simulink model "multi_rotor_sim"  (R2023b)
settings: Solver=ode4  StartTime=0.0  StopTime=inf  FixedStep=ST  RelTol=1e-3
values from neighbouring files (symbols this model uses):
  a0 = 0    [parameters.m]
  ASLOPE = 5.9    [parameters.m]
  Ax = 0.023    [parameters.m]
  Ay = 0.023    [parameters.m]
  Az = 0.106    [parameters.m]
  BLADES = 2    [parameters.m]
  BLCG = 0    [parameters.m]
  BLCP = 0    [parameters.m]
  BLH1 = b*sind(30)    [parameters.m]
  BLH2 = b    (= 0.275)    [parameters.m]
  BLH3 = b*sind(30)    [parameters.m]
  BLH4 = -b*sind(30)    [parameters.m]
  BLH5 = -b    (= -0.275)    [parameters.m]
  BLH6 = -b*sind(30)    [parameters.m]
  chi1 = 1    [parameters.m]
  chi2 = -1    [parameters.m]
  chi3 = 1    [parameters.m]
  chi4 = -1    [parameters.m]
  chi5 = 1    [parameters.m]
  chi6 = -1    [parameters.m]
  CHORD = 17.55e-3    (= 0.01755)    [parameters.m]
  CHORD75 = 21e-3    (= 0.021)    [parameters.m]
  dyn_viscosity = 17.89e-6    (= 1.789e-05)    [parameters.m]
  g0 = 9.80665    [parameters.m]
  href = 0    [parameters.m]
  k_ind = 1.35    [parameters.m]
  k_Omega = 14.92    [parameters.m]
  latref = 44.200626    [parameters.m]
  lonref = 12.063822    [parameters.m]
  m = 2.15    [parameters.m]
  MC_ATT_PITCH = 45*pi/180    (= 0.785398163397)    [parameters.m]
  MC_ATT_ROLL = 45*pi/180    (= 0.785398163397)    [parameters.m]
  MC_PITCH_P = 2    [parameters.m]
  MC_PITCHRATE_D = 0    [parameters.m]
  MC_PITCHRATE_I = 0.05    [parameters.m]
  MC_PITCHRATE_P = 0.09*3    (= 0.27)    [parameters.m]
  MC_RATE_PITCH = 500*pi/180    (= 8.72664625997)    [parameters.m]
  MC_RATE_ROLL = 500*pi/180    (= 8.72664625997)    [parameters.m]
  MC_RATE_YAW = 300*pi/180    (= 5.23598775598)    [parameters.m]
  MC_ROLL_P = 2    [parameters.m]
  MC_ROLLRATE_D = 0    [parameters.m]
  MC_ROLLRATE_I = 0.05    [parameters.m]
  MC_ROLLRATE_P = 0.09*3    (= 0.27)    [parameters.m]
  MC_VEL_FWD = 15    [parameters.m]
  MC_VEL_FWD_OPT = 0.5    [parameters.m]
  MC_VEL_LAT = 15    [parameters.m]
  MC_VEL_LAT_OPT = 0.5    [parameters.m]
  MC_VEL_VERT = 15    [parameters.m]
  MC_YAW_P = 0.55    [parameters.m]
  MC_YAWRATE_D = 0.05    [parameters.m]
  MC_YAWRATE_I = 0.02    [parameters.m]
  MC_YAWRATE_P = 0.15*3    (= 0.45)    [parameters.m]
  MPC_XY_VEL_D_ACC = 0.6    [parameters.m]
  MPC_XY_VEL_I_ACC = 0.8    [parameters.m]
  MPC_XY_VEL_P_ACC = 1.7    [parameters.m]
  MPC_Z_VEL_D_ACC = 0    [parameters.m]
  MPC_Z_VEL_I_ACC = 2    [parameters.m]
  MPC_Z_VEL_P_ACC = 4    [parameters.m]
  n = 0.6359    [parameters.m]
  p00 = 7.145e-2    (= 0.07145)    [parameters.m]
  p01 = 0.4377    [parameters.m]
  p02 = -10.13    [parameters.m]
  p10 = 1.259e-3    (= 0.001259)    [parameters.m]
  p11 = 1.284e-3    (= 0.001284)    [parameters.m]
  p20 = -7.513e-7    (= -7.513e-07)    [parameters.m]
  PWM_hover = (PWM_idle+PWM_max)/2    (= 1550)    [parameters.m]
  PWM_idle = 1100    [parameters.m]
  PWM_max = 2000    [parameters.m]
  ROTOR = 4*0.0254    (= 0.1016)    [parameters.m]
  ST = 0.01    [parameters.m]
  STACG = 0    [parameters.m]
  STACP = 0    [parameters.m]
  STAH1 = -b*cosd(30)    [parameters.m]
  STAH2 = 0    [parameters.m]
  STAH3 = b*cosd(30)    [parameters.m]
  STAH4 = b*cosd(30)    [parameters.m]
  STAH5 = 0    [parameters.m]
  STAH6 = -b*cosd(30)    [parameters.m]
  TERMINAL_SPEED = 0.5    [parameters.m]
  Theta0 = 45*pi/180    (= 0.785398163397)    [parameters.m]
  THETT = -38.0973*pi/180    (= -0.66492332112)    [parameters.m]
  wind_rate = [ 0 0 0 ]'    [parameters.m]
  wind_velocity_e = [ 0 0 0 ]'    [parameters.m]
  WLCG = -0.02    [parameters.m]
  WLCP = -0.08    [parameters.m]
  WLH1 = 32e-3    (= 0.032)    [parameters.m]
  WLH2 = 32e-3    (= 0.032)    [parameters.m]
  WLH3 = 32e-3    (= 0.032)    [parameters.m]
  WLH4 = 32e-3    (= 0.032)    [parameters.m]
  WLH5 = 32e-3    (= 0.032)    [parameters.m]
  WLH6 = 32e-3    (= 0.032)    [parameters.m]
undefined symbols (not defined in the file or in its folder): Earth, WGS84, X, Y, Z
libraries: sm_lib x258, slpidlib x36, nesl_utility x15, sharedtransform x13, aerolibutil x4, aerolibanimutils x3, sharedutil x2, sim3dlib x1, uavsim3dlib x1, shared6dof x1, aerolibtransform2 x1, aerolibatmos2 x1
(part 8 of 11)

== system multi_rotor_sim/3D_visualization/SIMECHANICS 3D SCENE/SimMechanics/MotorA/DCBL_Assembly_Clockwise_1_Top_1_RIGID ==
  Assem1DCBL_Assembly_Clockwise_1_Top_1_RIGID : Subsystem
  ReferenceFrame : sm_lib/Frames and Transforms/Reference Frame
  Transform : sm_lib/Frames and Transforms/Rigid Transform  TranslationMethod=Cartesian  TranslationStandardOffset=0  TranslationStandardOffsetUnits=mm  TranslationStandardAxis=+Z  TranslationCartesianOffset=[-1.7338900268269642e-14 5.4999999999999929 -2.252012665224854e-14]  TranslationCartesianOffsetUnits=mm  TranslationROffset=0  TranslationROffsetUnits=m  TranslationZOffset=0  TranslationZOffsetUnits=m  TranslationThetaOffset=0  TranslationThetaOffsetUnits=deg  RotationMethod=ArbitraryAxis  RotationAngleUnits=rad  RotationStandardAxis=+Z  RotationAngle=2.0943951023931957  RotationArbitraryAxis=[0.57735026918962584 -0.57735026918962573 0.57735026918962573]  FollAlignAxisA=+X  BaseAlignAxisA=+Y  FollAlignAxisB=+Y  BaseAlignAxisB=+Z  RotationSequenceAxes=FollowerAxes  RotationSequence=XYX  RotationSequenceAngles=[0 0 0]  RotationSequenceAnglesUnits=deg  RotationMatrix=[1 0 0; 0 1 0; 0 0 1]  Quaternion=[1 0 0 0]
  F : PMIOPort  Side=Left
  connections:
  ReferenceFrame/RConn1 -- Assem1DCBL_Assembly_Clockwise_1_Top_1_RIGID/LConn1 -- Transform/LConn1
  Transform/RConn1 -- F/RConn1

== system multi_rotor_sim/3D_visualization/SIMECHANICS 3D SCENE/SimMechanics/MotorB/DCBL_Assembly_CounterClockwise_2_Top_1_RIGID ==
  Assem2DCBL_Assembly_CounterClockwise_2_Top_1_RIGID : Subsystem
  ReferenceFrame : sm_lib/Frames and Transforms/Reference Frame
  Transform : sm_lib/Frames and Transforms/Rigid Transform  TranslationMethod=Cartesian  TranslationStandardOffset=0  TranslationStandardOffsetUnits=mm  TranslationStandardAxis=+Z  TranslationCartesianOffset=[5.4329271302963538e-14 5.5000000000000071 -8.6888702660306153e-14]  TranslationCartesianOffsetUnits=mm  TranslationROffset=0  TranslationROffsetUnits=m  TranslationZOffset=0  TranslationZOffsetUnits=m  TranslationThetaOffset=0  TranslationThetaOffsetUnits=deg  RotationMethod=ArbitraryAxis  RotationAngleUnits=rad  RotationStandardAxis=+Z  RotationAngle=2.0943951023931953  RotationArbitraryAxis=[0.57735026918962584 -0.57735026918962584 0.57735026918962584]  FollAlignAxisA=+X  BaseAlignAxisA=+Y  FollAlignAxisB=+Y  BaseAlignAxisB=+Z  RotationSequenceAxes=FollowerAxes  RotationSequence=XYX  RotationSequenceAngles=[0 0 0]  RotationSequenceAnglesUnits=deg  RotationMatrix=[1 0 0; 0 1 0; 0 0 1]  Quaternion=[1 0 0 0]
  F : PMIOPort  Side=Left
  connections:
  ReferenceFrame/RConn1 -- Assem2DCBL_Assembly_CounterClockwise_2_Top_1_RIGID/LConn1 -- Transform/LConn1
  Transform/RConn1 -- F/RConn1

== system multi_rotor_sim/3D_visualization/SIMECHANICS 3D SCENE/SimMechanics/MotorC/DCBL_Assembly_Clockwise_3_Top_1_RIGID ==
  Assem3DCBL_Assembly_Clockwise_3_Top_1_RIGID : Subsystem
  ReferenceFrame : sm_lib/Frames and Transforms/Reference Frame
  Transform : sm_lib/Frames and Transforms/Rigid Transform  TranslationMethod=Cartesian  TranslationStandardOffset=0  TranslationStandardOffsetUnits=mm  TranslationStandardAxis=+Z  TranslationCartesianOffset=[2.4199042072407481e-15 5.5000000000000071 -2.0095726513600741e-13]  TranslationCartesianOffsetUnits=mm  TranslationROffset=0  TranslationROffsetUnits=m  TranslationZOffset=0  TranslationZOffsetUnits=m  TranslationThetaOffset=0  TranslationThetaOffsetUnits=deg  RotationMethod=ArbitraryAxis  RotationAngleUnits=rad  RotationStandardAxis=+Z  RotationAngle=2.0943951023931953  RotationArbitraryAxis=[0.57735026918962584 -0.57735026918962584 0.57735026918962584]  FollAlignAxisA=+X  BaseAlignAxisA=+Y  FollAlignAxisB=+Y  BaseAlignAxisB=+Z  RotationSequenceAxes=FollowerAxes  RotationSequence=XYX  RotationSequenceAngles=[0 0 0]  RotationSequenceAnglesUnits=deg  RotationMatrix=[1 0 0; 0 1 0; 0 0 1]  Quaternion=[1 0 0 0]
  F : PMIOPort  Side=Left
  connections:
  ReferenceFrame/RConn1 -- Assem3DCBL_Assembly_Clockwise_3_Top_1_RIGID/LConn1 -- Transform/LConn1
  Transform/RConn1 -- F/RConn1

== system multi_rotor_sim/3D_visualization/SIMECHANICS 3D SCENE/SimMechanics/MotorD/DCBL_Assembly_CounterClockwise_4_Top_1_RIGID ==
  Assem4DCBL_Assembly_CounterClockwise_4_Top_1_RIGID : Subsystem
  ReferenceFrame : sm_lib/Frames and Transforms/Reference Frame
  Transform : sm_lib/Frames and Transforms/Rigid Transform  TranslationMethod=Cartesian  TranslationStandardOffset=0  TranslationStandardOffsetUnits=mm  TranslationStandardAxis=+Z  TranslationCartesianOffset=[2.4451512600426024e-14 5.5000000000000071 -1.4488516090253114e-14]  TranslationCartesianOffsetUnits=mm  TranslationROffset=0  TranslationROffsetUnits=m  TranslationZOffset=0  TranslationZOffsetUnits=m  TranslationThetaOffset=0  TranslationThetaOffsetUnits=deg  RotationMethod=ArbitraryAxis  RotationAngleUnits=rad  RotationStandardAxis=+Z  RotationAngle=2.0943951023931953  RotationArbitraryAxis=[0.57735026918962584 -0.57735026918962584 0.57735026918962584]  FollAlignAxisA=+X  BaseAlignAxisA=+Y  FollAlignAxisB=+Y  BaseAlignAxisB=+Z  RotationSequenceAxes=FollowerAxes  RotationSequence=XYX  RotationSequenceAngles=[0 0 0]  RotationSequenceAnglesUnits=deg  RotationMatrix=[1 0 0; 0 1 0; 0 0 1]  Quaternion=[1 0 0 0]
  F : PMIOPort  Side=Left
  connections:
  ReferenceFrame/RConn1 -- Assem4DCBL_Assembly_CounterClockwise_4_Top_1_RIGID/LConn1 -- Transform/LConn1
  Transform/RConn1 -- F/RConn1

== system multi_rotor_sim/3D_visualization/SIMECHANICS 3D SCENE/SimMechanics/Assembly_Quadrotor_NProp_1_RIGID/Assembly_Quadrotor_NoProp_1_RIGID/Arm1_DJI_F450_F550_Final_2_RIGID ==
  ReferenceFrame : sm_lib/Frames and Transforms/Reference Frame
  Solid : sm_lib/Body Elements/File Solid  ExtGeomFileName=Arm1-DJI F450 F550_Final_Default_sldprt.STL  UnitType=Custom  ExtGeomFileUnits=mm  StepReaderType=HEX  ExportConvexHullGeometry=off  InertiaType=Custom  Mass=0.040949498799243353  MassUnits=kg  CenterOfMass=[91.850565621128027 -9.6558313898433461 0.00059254732510302048]  CenterOfMassUnits=mm  MomentsOfInertia=[8.7857917451793011 208.43528107693191 210.30930845149899]  MomentsOfInertiaUnits=kg*mm^2  ProductsOfInertia=[0.00021379289914309399 -0.0030630676058125863 -5.324939120360261]  ProductsOfInertiaUnits=kg*mm^2  BasedOnType=Density  Density=1000  DensityUnits=kg/(m^3)  DoExposeReferenceFrame=on  SerializedFrames=<Frames/>  GraphicType=FromGeometry  MarkerShape=Sphere  MarkerSize=10  MarkerSizeUnits=m  GraphicVisPropType=SimpleVisualProperties  GraphicDiffuseColor=[1 1 1]  GraphicSpecularColor=[0.5 0.5 0.5 1.0]  GraphicAmbientColor=[0.15 0.15 0.15 1.0]  GraphicEmissiveColor=[0.0 0.0 0.0 1.0]  GraphicShininess=75  GraphicOpacity=1
  F : PMIOPort  Side=Left
  connections:
  Solid/RConn1 -- ReferenceFrame/RConn1 -- F/RConn1

== system multi_rotor_sim/3D_visualization/SIMECHANICS 3D SCENE/SimMechanics/Assembly_Quadrotor_NProp_1_RIGID/Assembly_Quadrotor_NoProp_1_RIGID/ArmRed1_DJI_F450_F550_Final_1_RIGID ==
  ReferenceFrame : sm_lib/Frames and Transforms/Reference Frame
  Solid : sm_lib/Body Elements/File Solid  ExtGeomFileName=ArmRed1-DJI F450 F550_Final_Default_sldprt.STL  UnitType=Custom  ExtGeomFileUnits=mm  StepReaderType=HEX  ExportConvexHullGeometry=off  InertiaType=Custom  Mass=0.040949498799243353  MassUnits=kg  CenterOfMass=[91.850565621128027 -9.6558313898433408 0.00059254732510311101]  CenterOfMassUnits=mm  MomentsOfInertia=[8.7857917451792904 208.43528107693191 210.30930845149899]  MomentsOfInertiaUnits=kg*mm^2  ProductsOfInertia=[0.00021379289914303225 -0.0030630676058125412 -5.3249391203602654]  ProductsOfInertiaUnits=kg*mm^2  BasedOnType=Density  Density=1000  DensityUnits=kg/(m^3)  DoExposeReferenceFrame=on  SerializedFrames=<Frames/>  GraphicType=FromGeometry  MarkerShape=Sphere  MarkerSize=10  MarkerSizeUnits=m  GraphicVisPropType=SimpleVisualProperties  GraphicDiffuseColor=[0.0 0.0 0.8]  GraphicSpecularColor=[0.5 0.5 0.5 1.0]  GraphicAmbientColor=[0.15 0.15 0.15 1.0]  GraphicEmissiveColor=[0.0 0.0 0.0 1.0]  GraphicShininess=75  GraphicOpacity=1
  F : PMIOPort  Side=Left
  connections:
  Solid/RConn1 -- ReferenceFrame/RConn1 -- F/RConn1

== system multi_rotor_sim/3D_visualization/SIMECHANICS 3D SCENE/SimMechanics/Assembly_Quadrotor_NProp_1_RIGID/Assembly_Quadrotor_NoProp_1_RIGID/ArmRed_DJI_F450_F550_Final_1_RIGID ==
  ReferenceFrame : sm_lib/Frames and Transforms/Reference Frame
  Solid : sm_lib/Body Elements/File Solid  ExtGeomFileName=ArmRed-DJI F450 F550_Final_Default_sldprt.STL  UnitType=Custom  ExtGeomFileUnits=mm  StepReaderType=HEX  ExportConvexHullGeometry=off  InertiaType=Custom  Mass=0.040949498799243353  MassUnits=kg  CenterOfMass=[91.850565621128027 -9.6558313898433461 0.00059254732510311101]  CenterOfMassUnits=mm  MomentsOfInertia=[8.7857917451793011 208.43528107693191 210.30930845149899]  MomentsOfInertiaUnits=kg*mm^2  ProductsOfInertia=[0.00021379289914314785 -0.0030630676058125421 -5.3249391203602672]  ProductsOfInertiaUnits=kg*mm^2  BasedOnType=Density  Density=1000  DensityUnits=kg/(m^3)  DoExposeReferenceFrame=on  SerializedFrames=<Frames/>  GraphicType=FromGeometry  MarkerShape=Sphere  MarkerSize=10  MarkerSizeUnits=m  GraphicVisPropType=SimpleVisualProperties  GraphicDiffuseColor=[0.0 0.0 0.8]  GraphicSpecularColor=[0.5 0.5 0.5 1.0]  GraphicAmbientColor=[0.15 0.15 0.15 1.0]  GraphicEmissiveColor=[0.0 0.0 0.0 1.0]  GraphicShininess=75  GraphicOpacity=1
  F : PMIOPort  Side=Left
  connections:
  Solid/RConn1 -- ReferenceFrame/RConn1 -- F/RConn1

== system multi_rotor_sim/3D_visualization/SIMECHANICS 3D SCENE/SimMechanics/Assembly_Quadrotor_NProp_1_RIGID/Assembly_Quadrotor_NoProp_1_RIGID/Arm_DJI_F450_F550_Final_1_RIGID ==
  ReferenceFrame : sm_lib/Frames and Transforms/Reference Frame
  Solid : sm_lib/Body Elements/File Solid  ExtGeomFileName=Arm-DJI F450 F550_Final_Default_sldprt.STL  UnitType=Custom  ExtGeomFileUnits=mm  StepReaderType=HEX  ExportConvexHullGeometry=off  InertiaType=Custom  Mass=0.040949498799243353  MassUnits=kg  CenterOfMass=[91.850565621128027 -9.6558313898433461 0.00059254732510274899]  CenterOfMassUnits=mm  MomentsOfInertia=[8.7857917451793011 208.43528107693191 210.30930845149899]  MomentsOfInertiaUnits=kg*mm^2  ProductsOfInertia=[0.00021379289914293239 -0.0030630676058130682 -5.324939120360269]  ProductsOfInertiaUnits=kg*mm^2  BasedOnType=Density  Density=1000  DensityUnits=kg/(m^3)  DoExposeReferenceFrame=on  SerializedFrames=<Frames/>  GraphicType=FromGeometry  MarkerShape=Sphere  MarkerSize=10  MarkerSizeUnits=m  GraphicVisPropType=SimpleVisualProperties  GraphicDiffuseColor=[1 1 1]  GraphicSpecularColor=[0.5 0.5 0.5 1.0]  GraphicAmbientColor=[0.15 0.15 0.15 1.0]  GraphicEmissiveColor=[0.0 0.0 0.0 1.0]  GraphicShininess=75  GraphicOpacity=1
  F : PMIOPort  Side=Left
  connections:
  Solid/RConn1 -- ReferenceFrame/RConn1 -- F/RConn1

== system multi_rotor_sim/3D_visualization/SIMECHANICS 3D SCENE/SimMechanics/Assembly_Quadrotor_NProp_1_RIGID/Assembly_Quadrotor_NoProp_1_RIGID/Bottom_board_DJI_F450_Final_1_RIGID ==
  ReferenceFrame : sm_lib/Frames and Transforms/Reference Frame
  Solid : sm_lib/Body Elements/File Solid  ExtGeomFileName=Bottom board-DJI F450_Final_Default_sldprt.STL  UnitType=Custom  ExtGeomFileUnits=mm  StepReaderType=HEX  ExportConvexHullGeometry=off  InertiaType=Custom  Mass=0.022402083580285712  MassUnits=kg  CenterOfMass=[0 4.8087280328776543e-11 0]  CenterOfMassUnits=mm  MomentsOfInertia=[17.621231604317398 65.326748791856005 47.714143483190369]  MomentsOfInertiaUnits=kg*mm^2  ProductsOfInertia=[0 0 0]  ProductsOfInertiaUnits=kg*mm^2  BasedOnType=Density  Density=1000  DensityUnits=kg/(m^3)  DoExposeReferenceFrame=on  SerializedFrames=<Frames/>  GraphicType=FromGeometry  MarkerShape=Sphere  MarkerSize=10  MarkerSizeUnits=m  GraphicVisPropType=SimpleVisualProperties  GraphicDiffuseColor=[0 0 0]  GraphicSpecularColor=[0.5 0.5 0.5 1.0]  GraphicAmbientColor=[0.15 0.15 0.15 1.0]  GraphicEmissiveColor=[0.0 0.0 0.0 1.0]  GraphicShininess=75  GraphicOpacity=1
  F : PMIOPort  Side=Left
  connections:
  Solid/RConn1 -- ReferenceFrame/RConn1 -- F/RConn1

== system multi_rotor_sim/3D_visualization/SIMECHANICS 3D SCENE/SimMechanics/Assembly_Quadrotor_NProp_1_RIGID/Assembly_Quadrotor_NoProp_1_RIGID/DCBL_Assembly_Clockwise_1_Bottom_1_RIGID ==
  De_DCBL_1_RIGID : Subsystem
  ReferenceFrame : sm_lib/Frames and Transforms/Reference Frame
  Transform : sm_lib/Frames and Transforms/Rigid Transform  TranslationMethod=None  TranslationStandardOffset=0  TranslationStandardOffsetUnits=m  TranslationStandardAxis=+Z  TranslationCartesianOffset=[0 0 0]  TranslationCartesianOffsetUnits=m  TranslationROffset=0  TranslationROffsetUnits=m  TranslationZOffset=0  TranslationZOffsetUnits=m  TranslationThetaOffset=0  TranslationThetaOffsetUnits=deg  RotationMethod=None  RotationAngleUnits=deg  RotationStandardAxis=+Z  RotationAngle=0  RotationArbitraryAxis=[0 0 1]  FollAlignAxisA=+X  BaseAlignAxisA=+Y  FollAlignAxisB=+Y  BaseAlignAxisB=+Z  RotationSequenceAxes=FollowerAxes  RotationSequence=XYX  RotationSequenceAngles=[0 0 0]  RotationSequenceAnglesUnits=deg  RotationMatrix=[1 0 0; 0 1 0; 0 0 1]  Quaternion=[1 0 0 0]
  Transform1 : sm_lib/Frames and Transforms/Rigid Transform  TranslationMethod=Cartesian  TranslationStandardOffset=0  TranslationStandardOffsetUnits=mm  TranslationStandardAxis=+Z  TranslationCartesianOffset=[159.70006653098284 35.76000000009617 159.70006653098039]  TranslationCartesianOffsetUnits=mm  TranslationROffset=0  TranslationROffsetUnits=m  TranslationZOffset=0  TranslationZOffsetUnits=m  TranslationThetaOffset=0  TranslationThetaOffsetUnits=deg  RotationMethod=ArbitraryAxis  RotationAngleUnits=rad  RotationStandardAxis=+Z  RotationAngle=0.78539816339744029  RotationArbitraryAxis=[0 -1 0]  FollAlignAxisA=+X  BaseAlignAxisA=+Y  FollAlignAxisB=+Y  BaseAlignAxisB=+Z  RotationSequenceAxes=FollowerAxes  RotationSequence=XYX  RotationSequenceAngles=[0 0 0]  RotationSequenceAnglesUnits=deg  RotationMatrix=[1 0 0; 0 1 0; 0 0 1]  Quaternion=[1 0 0 0]
  F : PMIOPort  Side=Right
  connections:
  De_DCBL_1_RIGID/LConn1 -- Transform/RConn1
  Transform/LConn1 -- ReferenceFrame/RConn1 -- Transform1/RConn1
  Transform1/LConn1 -- F/RConn1

== system multi_rotor_sim/3D_visualization/SIMECHANICS 3D SCENE/SimMechanics/Assembly_Quadrotor_NProp_1_RIGID/Assembly_Quadrotor_NoProp_1_RIGID/DCBL_Assembly_Clockwise_3_Bottom_1_RIGID ==
  De_DCBL_1_RIGID : Subsystem
  ReferenceFrame : sm_lib/Frames and Transforms/Reference Frame
  Transform : sm_lib/Frames and Transforms/Rigid Transform  TranslationMethod=None  TranslationStandardOffset=0  TranslationStandardOffsetUnits=m  TranslationStandardAxis=+Z  TranslationCartesianOffset=[0 0 0]  TranslationCartesianOffsetUnits=m  TranslationROffset=0  TranslationROffsetUnits=m  TranslationZOffset=0  TranslationZOffsetUnits=m  TranslationThetaOffset=0  TranslationThetaOffsetUnits=deg  RotationMethod=None  RotationAngleUnits=deg  RotationStandardAxis=+Z  RotationAngle=0  RotationArbitraryAxis=[0 0 1]  FollAlignAxisA=+X  BaseAlignAxisA=+Y  FollAlignAxisB=+Y  BaseAlignAxisB=+Z  RotationSequenceAxes=FollowerAxes  RotationSequence=XYX  RotationSequenceAngles=[0 0 0]  RotationSequenceAnglesUnits=deg  RotationMatrix=[1 0 0; 0 1 0; 0 0 1]  Quaternion=[1 0 0 0]
  Transform1 : sm_lib/Frames and Transforms/Rigid Transform  TranslationMethod=Cartesian  TranslationStandardOffset=0  TranslationStandardOffsetUnits=mm  TranslationStandardAxis=+Z  TranslationCartesianOffset=[-159.70006653098244 35.76000000009617 -159.70006653098108]  TranslationCartesianOffsetUnits=mm  TranslationROffset=0  TranslationROffsetUnits=m  TranslationZOffset=0  TranslationZOffsetUnits=m  TranslationThetaOffset=0  TranslationThetaOffsetUnits=deg  RotationMethod=ArbitraryAxis  RotationAngleUnits=rad  RotationStandardAxis=+Z  RotationAngle=0.78539816339744262  RotationArbitraryAxis=[0 -1 0]  FollAlignAxisA=+X  BaseAlignAxisA=+Y  FollAlignAxisB=+Y  BaseAlignAxisB=+Z  RotationSequenceAxes=FollowerAxes  RotationSequence=XYX  RotationSequenceAngles=[0 0 0]  RotationSequenceAnglesUnits=deg  RotationMatrix=[1 0 0; 0 1 0; 0 0 1]  Quaternion=[1 0 0 0]
  F : PMIOPort  Side=Right
  connections:
  De_DCBL_1_RIGID/LConn1 -- Transform/RConn1
  Transform/LConn1 -- ReferenceFrame/RConn1 -- Transform1/RConn1
  Transform1/LConn1 -- F/RConn1

== system multi_rotor_sim/3D_visualization/SIMECHANICS 3D SCENE/SimMechanics/Assembly_Quadrotor_NProp_1_RIGID/Assembly_Quadrotor_NoProp_1_RIGID/DCBL_Assembly_CounterClockwise_2_Bottom_1_RIGID ==
  De_DCBL_1_RIGID : Subsystem
  ReferenceFrame : sm_lib/Frames and Transforms/Reference Frame
  Transform : sm_lib/Frames and Transforms/Rigid Transform  TranslationMethod=None  TranslationStandardOffset=0  TranslationStandardOffsetUnits=m  TranslationStandardAxis=+Z  TranslationCartesianOffset=[0 0 0]  TranslationCartesianOffsetUnits=m  TranslationROffset=0  TranslationROffsetUnits=m  TranslationZOffset=0  TranslationZOffsetUnits=m  TranslationThetaOffset=0  TranslationThetaOffsetUnits=deg  RotationMethod=None  RotationAngleUnits=deg  RotationStandardAxis=+Z  RotationAngle=0  RotationArbitraryAxis=[0 0 1]  FollAlignAxisA=+X  BaseAlignAxisA=+Y  FollAlignAxisB=+Y  BaseAlignAxisB=+Z  RotationSequenceAxes=FollowerAxes  RotationSequence=XYX  RotationSequenceAngles=[0 0 0]  RotationSequenceAnglesUnits=deg  RotationMatrix=[1 0 0; 0 1 0; 0 0 1]  Quaternion=[1 0 0 0]
  Transform1 : sm_lib/Frames and Transforms/Rigid Transform  TranslationMethod=Cartesian  TranslationStandardOffset=0  TranslationStandardOffsetUnits=mm  TranslationStandardAxis=+Z  TranslationCartesianOffset=[159.7000665309815 35.76000000009617 -159.70006653098207]  TranslationCartesianOffsetUnits=mm  TranslationROffset=0  TranslationROffsetUnits=m  TranslationZOffset=0  TranslationZOffsetUnits=m  TranslationThetaOffset=0  TranslationThetaOffsetUnits=deg  RotationMethod=ArbitraryAxis  RotationAngleUnits=rad  RotationStandardAxis=+Z  RotationAngle=0.78539816339744961  RotationArbitraryAxis=[0 1 0]  FollAlignAxisA=+X  BaseAlignAxisA=+Y  FollAlignAxisB=+Y  BaseAlignAxisB=+Z  RotationSequenceAxes=FollowerAxes  RotationSequence=XYX  RotationSequenceAngles=[0 0 0]  RotationSequenceAnglesUnits=deg  RotationMatrix=[1 0 0; 0 1 0; 0 0 1]  Quaternion=[1 0 0 0]
  F : PMIOPort  Side=Right
  connections:
  De_DCBL_1_RIGID/LConn1 -- Transform/RConn1
  Transform/LConn1 -- ReferenceFrame/RConn1 -- Transform1/RConn1
  Transform1/LConn1 -- F/RConn1

== system multi_rotor_sim/3D_visualization/SIMECHANICS 3D SCENE/SimMechanics/Assembly_Quadrotor_NProp_1_RIGID/Assembly_Quadrotor_NoProp_1_RIGID/DCBL_Assembly_CounterClockwise_4_Bottom_1_RIGID ==
  De_DCBL_1_RIGID : Subsystem
  ReferenceFrame : sm_lib/Frames and Transforms/Reference Frame
  Transform : sm_lib/Frames and Transforms/Rigid Transform  TranslationMethod=None  TranslationStandardOffset=0  TranslationStandardOffsetUnits=m  TranslationStandardAxis=+Z  TranslationCartesianOffset=[0 0 0]  TranslationCartesianOffsetUnits=m  TranslationROffset=0  TranslationROffsetUnits=m  TranslationZOffset=0  TranslationZOffsetUnits=m  TranslationThetaOffset=0  TranslationThetaOffsetUnits=deg  RotationMethod=None  RotationAngleUnits=deg  RotationStandardAxis=+Z  RotationAngle=0  RotationArbitraryAxis=[0 0 1]  FollAlignAxisA=+X  BaseAlignAxisA=+Y  FollAlignAxisB=+Y  BaseAlignAxisB=+Z  RotationSequenceAxes=FollowerAxes  RotationSequence=XYX  RotationSequenceAngles=[0 0 0]  RotationSequenceAnglesUnits=deg  RotationMatrix=[1 0 0; 0 1 0; 0 0 1]  Quaternion=[1 0 0 0]
  Transform1 : sm_lib/Frames and Transforms/Rigid Transform  TranslationMethod=Cartesian  TranslationStandardOffset=0  TranslationStandardOffsetUnits=mm  TranslationStandardAxis=+Z  TranslationCartesianOffset=[-159.70006653098127 35.76000000009617 159.70006653098196]  TranslationCartesianOffsetUnits=mm  TranslationROffset=0  TranslationROffsetUnits=m  TranslationZOffset=0  TranslationZOffsetUnits=m  TranslationThetaOffset=0  TranslationThetaOffsetUnits=deg  RotationMethod=ArbitraryAxis  RotationAngleUnits=rad  RotationStandardAxis=+Z  RotationAngle=0.78539816339745094  RotationArbitraryAxis=[0 1 0]  FollAlignAxisA=+X  BaseAlignAxisA=+Y  FollAlignAxisB=+Y  BaseAlignAxisB=+Z  RotationSequenceAxes=FollowerAxes  RotationSequence=XYX  RotationSequenceAngles=[0 0 0]  RotationSequenceAnglesUnits=deg  RotationMatrix=[1 0 0; 0 1 0; 0 0 1]  Quaternion=[1 0 0 0]
  F : PMIOPort  Side=Right
  connections:
  De_DCBL_1_RIGID/LConn1 -- Transform/RConn1
  Transform/LConn1 -- ReferenceFrame/RConn1 -- Transform1/RConn1
  Transform1/LConn1 -- F/RConn1

== system multi_rotor_sim/3D_visualization/SIMECHANICS 3D SCENE/SimMechanics/Assembly_Quadrotor_NProp_1_RIGID/Assembly_Quadrotor_NoProp_1_RIGID/Top_board_DJI_F450_Final_1_RIGID ==
  ReferenceFrame : sm_lib/Frames and Transforms/Reference Frame
  Solid : sm_lib/Body Elements/File Solid  ExtGeomFileName=Top board-DJI F450_Final_Default_sldprt.STL  UnitType=Custom  ExtGeomFileUnits=mm  StepReaderType=HEX  ExportConvexHullGeometry=off  InertiaType=Custom  Mass=0.013626610836899209  MassUnits=kg  CenterOfMass=[0 0 0]  CenterOfMassUnits=mm  MomentsOfInertia=[11.678434060128888 23.780162168623775 12.106975262107815]  MomentsOfInertiaUnits=kg*mm^2  ProductsOfInertia=[0 0 0]  ProductsOfInertiaUnits=kg*mm^2  BasedOnType=Density  Density=1000  DensityUnits=kg/(m^3)  DoExposeReferenceFrame=on  SerializedFrames=<Frames/>  GraphicType=FromGeometry  MarkerShape=Sphere  MarkerSize=10  MarkerSizeUnits=m  GraphicVisPropType=SimpleVisualProperties  GraphicDiffuseColor=[0 0 0]  GraphicSpecularColor=[0.5 0.5 0.5 1.0]  GraphicAmbientColor=[0.15 0.15 0.15 1.0]  GraphicEmissiveColor=[0.0 0.0 0.0 1.0]  GraphicShininess=75  GraphicOpacity=1
  F : PMIOPort  Side=Left
  connections:
  Solid/RConn1 -- ReferenceFrame/RConn1 -- F/RConn1

== system multi_rotor_sim/3D_visualization/SIMECHANICS 3D SCENE/SimMechanics/Assembly_Quadrotor_NProp_1_RIGID/Assembly_Quadrotor_NoProp_1_RIGID/socket_head_cap_screw_iso_10_RIGID ==
  ReferenceFrame : sm_lib/Frames and Transforms/Reference Frame
  Solid : sm_lib/Body Elements/File Solid  ExtGeomFileName=socket head cap screw_iso_ISO 4762 M3 x 5 --- 5N_sldprt.STL  UnitType=Custom  ExtGeomFileUnits=mm  StepReaderType=HEX  ExportConvexHullGeometry=off  InertiaType=Custom  Mass=9.7562055451047927e-05  MassUnits=kg  CenterOfMass=[2.9922591429378405 0 0]  CenterOfMassUnits=mm  MomentsOfInertia=[0.00030067681878230242 0.000604867911685519 0.00060486791168551911]  MomentsOfInertiaUnits=kg*mm^2  ProductsOfInertia=[0 0 0]  ProductsOfInertiaUnits=kg*mm^2  BasedOnType=Density  Density=1000  DensityUnits=kg/(m^3)  DoExposeReferenceFrame=on  SerializedFrames=<Frames/>  GraphicType=FromGeometry  MarkerShape=Sphere  MarkerSize=10  MarkerSizeUnits=m  GraphicVisPropType=SimpleVisualProperties  GraphicDiffuseColor=[0.77647058823529413 0.75686274509803919 0.73725490196078436]  GraphicSpecularColor=[0.5 0.5 0.5 1.0]  GraphicAmbientColor=[0.15 0.15 0.15 1.0]  GraphicEmissiveColor=[0.0 0.0 0.0 1.0]  GraphicShininess=75  GraphicOpacity=1
  F : PMIOPort  Side=Left
  connections:
  Solid/RConn1 -- ReferenceFrame/RConn1 -- F/RConn1

== system multi_rotor_sim/3D_visualization/SIMECHANICS 3D SCENE/SimMechanics/Assembly_Quadrotor_NProp_1_RIGID/Assembly_Quadrotor_NoProp_1_RIGID/socket_head_cap_screw_iso_11_RIGID ==
  ReferenceFrame : sm_lib/Frames and Transforms/Reference Frame
  Solid : sm_lib/Body Elements/File Solid  ExtGeomFileName=socket head cap screw_iso_ISO 4762 M3 x 5 --- 5N_sldprt.STL  UnitType=Custom  ExtGeomFileUnits=mm  StepReaderType=HEX  ExportConvexHullGeometry=off  InertiaType=Custom  Mass=9.7562055451047927e-05  MassUnits=kg  CenterOfMass=[2.9922591429378405 0 0]  CenterOfMassUnits=mm  MomentsOfInertia=[0.00030067681878230242 0.000604867911685519 0.00060486791168551911]  MomentsOfInertiaUnits=kg*mm^2  ProductsOfInertia=[0 0 0]  ProductsOfInertiaUnits=kg*mm^2  BasedOnType=Density  Density=1000  DensityUnits=kg/(m^3)  DoExposeReferenceFrame=on  SerializedFrames=<Frames/>  GraphicType=FromGeometry  MarkerShape=Sphere  MarkerSize=10  MarkerSizeUnits=m  GraphicVisPropType=SimpleVisualProperties  GraphicDiffuseColor=[0.77647058823529413 0.75686274509803919 0.73725490196078436]  GraphicSpecularColor=[0.5 0.5 0.5 1.0]  GraphicAmbientColor=[0.15 0.15 0.15 1.0]  GraphicEmissiveColor=[0.0 0.0 0.0 1.0]  GraphicShininess=75  GraphicOpacity=1
  F : PMIOPort  Side=Left
  connections:
  Solid/RConn1 -- ReferenceFrame/RConn1 -- F/RConn1

== system multi_rotor_sim/3D_visualization/SIMECHANICS 3D SCENE/SimMechanics/Assembly_Quadrotor_NProp_1_RIGID/Assembly_Quadrotor_NoProp_1_RIGID/socket_head_cap_screw_iso_12_RIGID ==
  ReferenceFrame : sm_lib/Frames and Transforms/Reference Frame
  Solid : sm_lib/Body Elements/File Solid  ExtGeomFileName=socket head cap screw_iso_ISO 4762 M3 x 5 --- 5N_sldprt.STL  UnitType=Custom  ExtGeomFileUnits=mm  StepReaderType=HEX  ExportConvexHullGeometry=off  InertiaType=Custom  Mass=9.7562055451047927e-05  MassUnits=kg  CenterOfMass=[2.9922591429378405 0 0]  CenterOfMassUnits=mm  MomentsOfInertia=[0.00030067681878230242 0.000604867911685519 0.00060486791168551911]  MomentsOfInertiaUnits=kg*mm^2  ProductsOfInertia=[0 0 0]  ProductsOfInertiaUnits=kg*mm^2  BasedOnType=Density  Density=1000  DensityUnits=kg/(m^3)  DoExposeReferenceFrame=on  SerializedFrames=<Frames/>  GraphicType=FromGeometry  MarkerShape=Sphere  MarkerSize=10  MarkerSizeUnits=m  GraphicVisPropType=SimpleVisualProperties  GraphicDiffuseColor=[0.77647058823529413 0.75686274509803919 0.73725490196078436]  GraphicSpecularColor=[0.5 0.5 0.5 1.0]  GraphicAmbientColor=[0.15 0.15 0.15 1.0]  GraphicEmissiveColor=[0.0 0.0 0.0 1.0]  GraphicShininess=75  GraphicOpacity=1
  F : PMIOPort  Side=Left
  connections:
  Solid/RConn1 -- ReferenceFrame/RConn1 -- F/RConn1

== system multi_rotor_sim/3D_visualization/SIMECHANICS 3D SCENE/SimMechanics/Assembly_Quadrotor_NProp_1_RIGID/Assembly_Quadrotor_NoProp_1_RIGID/socket_head_cap_screw_iso_13_RIGID ==
  ReferenceFrame : sm_lib/Frames and Transforms/Reference Frame
  Solid : sm_lib/Body Elements/File Solid  ExtGeomFileName=socket head cap screw_iso_ISO 4762 M3 x 5 --- 5N_sldprt.STL  UnitType=Custom  ExtGeomFileUnits=mm  StepReaderType=HEX  ExportConvexHullGeometry=off  InertiaType=Custom  Mass=9.7562055451047927e-05  MassUnits=kg  CenterOfMass=[2.9922591429378405 0 0]  CenterOfMassUnits=mm  MomentsOfInertia=[0.00030067681878230242 0.000604867911685519 0.00060486791168551911]  MomentsOfInertiaUnits=kg*mm^2  ProductsOfInertia=[0 0 0]  ProductsOfInertiaUnits=kg*mm^2  BasedOnType=Density  Density=1000  DensityUnits=kg/(m^3)  DoExposeReferenceFrame=on  SerializedFrames=<Frames/>  GraphicType=FromGeometry  MarkerShape=Sphere  MarkerSize=10  MarkerSizeUnits=m  GraphicVisPropType=SimpleVisualProperties  GraphicDiffuseColor=[0.77647058823529413 0.75686274509803919 0.73725490196078436]  GraphicSpecularColor=[0.5 0.5 0.5 1.0]  GraphicAmbientColor=[0.15 0.15 0.15 1.0]  GraphicEmissiveColor=[0.0 0.0 0.0 1.0]  GraphicShininess=75  GraphicOpacity=1
  F : PMIOPort  Side=Left
  connections:
  Solid/RConn1 -- ReferenceFrame/RConn1 -- F/RConn1

== system multi_rotor_sim/3D_visualization/SIMECHANICS 3D SCENE/SimMechanics/Assembly_Quadrotor_NProp_1_RIGID/Assembly_Quadrotor_NoProp_1_RIGID/socket_head_cap_screw_iso_14_RIGID ==
  ReferenceFrame : sm_lib/Frames and Transforms/Reference Frame
  Solid : sm_lib/Body Elements/File Solid  ExtGeomFileName=socket head cap screw_iso_ISO 4762 M3 x 5 --- 5N_sldprt.STL  UnitType=Custom  ExtGeomFileUnits=mm  StepReaderType=HEX  ExportConvexHullGeometry=off  InertiaType=Custom  Mass=9.7562055451047927e-05  MassUnits=kg  CenterOfMass=[2.9922591429378405 0 0]  CenterOfMassUnits=mm  MomentsOfInertia=[0.00030067681878230242 0.000604867911685519 0.00060486791168551911]  MomentsOfInertiaUnits=kg*mm^2  ProductsOfInertia=[0 0 0]  ProductsOfInertiaUnits=kg*mm^2  BasedOnType=Density  Density=1000  DensityUnits=kg/(m^3)  DoExposeReferenceFrame=on  SerializedFrames=<Frames/>  GraphicType=FromGeometry  MarkerShape=Sphere  MarkerSize=10  MarkerSizeUnits=m  GraphicVisPropType=SimpleVisualProperties  GraphicDiffuseColor=[0.77647058823529413 0.75686274509803919 0.73725490196078436]  GraphicSpecularColor=[0.5 0.5 0.5 1.0]  GraphicAmbientColor=[0.15 0.15 0.15 1.0]  GraphicEmissiveColor=[0.0 0.0 0.0 1.0]  GraphicShininess=75  GraphicOpacity=1
  F : PMIOPort  Side=Left
  connections:
  Solid/RConn1 -- ReferenceFrame/RConn1 -- F/RConn1

== system multi_rotor_sim/3D_visualization/SIMECHANICS 3D SCENE/SimMechanics/Assembly_Quadrotor_NProp_1_RIGID/Assembly_Quadrotor_NoProp_1_RIGID/socket_head_cap_screw_iso_15_RIGID ==
  ReferenceFrame : sm_lib/Frames and Transforms/Reference Frame
  Solid : sm_lib/Body Elements/File Solid  ExtGeomFileName=socket head cap screw_iso_ISO 4762 M3 x 5 --- 5N_sldprt.STL  UnitType=Custom  ExtGeomFileUnits=mm  StepReaderType=HEX  ExportConvexHullGeometry=off  InertiaType=Custom  Mass=9.7562055451047927e-05  MassUnits=kg  CenterOfMass=[2.9922591429378405 0 0]  CenterOfMassUnits=mm  MomentsOfInertia=[0.00030067681878230242 0.000604867911685519 0.00060486791168551911]  MomentsOfInertiaUnits=kg*mm^2  ProductsOfInertia=[0 0 0]  ProductsOfInertiaUnits=kg*mm^2  BasedOnType=Density  Density=1000  DensityUnits=kg/(m^3)  DoExposeReferenceFrame=on  SerializedFrames=<Frames/>  GraphicType=FromGeometry  MarkerShape=Sphere  MarkerSize=10  MarkerSizeUnits=m  GraphicVisPropType=SimpleVisualProperties  GraphicDiffuseColor=[0.77647058823529413 0.75686274509803919 0.73725490196078436]  GraphicSpecularColor=[0.5 0.5 0.5 1.0]  GraphicAmbientColor=[0.15 0.15 0.15 1.0]  GraphicEmissiveColor=[0.0 0.0 0.0 1.0]  GraphicShininess=75  GraphicOpacity=1
  F : PMIOPort  Side=Left
  connections:
  Solid/RConn1 -- ReferenceFrame/RConn1 -- F/RConn1

== system multi_rotor_sim/3D_visualization/SIMECHANICS 3D SCENE/SimMechanics/Assembly_Quadrotor_NProp_1_RIGID/Assembly_Quadrotor_NoProp_1_RIGID/socket_head_cap_screw_iso_16_RIGID ==
  ReferenceFrame : sm_lib/Frames and Transforms/Reference Frame
  Solid : sm_lib/Body Elements/File Solid  ExtGeomFileName=socket head cap screw_iso_ISO 4762 M3 x 5 --- 5N_sldprt.STL  UnitType=Custom  ExtGeomFileUnits=mm  StepReaderType=HEX  ExportConvexHullGeometry=off  InertiaType=Custom  Mass=9.7562055451047927e-05  MassUnits=kg  CenterOfMass=[2.9922591429378405 0 0]  CenterOfMassUnits=mm  MomentsOfInertia=[0.00030067681878230242 0.000604867911685519 0.00060486791168551911]  MomentsOfInertiaUnits=kg*mm^2  ProductsOfInertia=[0 0 0]  ProductsOfInertiaUnits=kg*mm^2  BasedOnType=Density  Density=1000  DensityUnits=kg/(m^3)  DoExposeReferenceFrame=on  SerializedFrames=<Frames/>  GraphicType=FromGeometry  MarkerShape=Sphere  MarkerSize=10  MarkerSizeUnits=m  GraphicVisPropType=SimpleVisualProperties  GraphicDiffuseColor=[0.77647058823529413 0.75686274509803919 0.73725490196078436]  GraphicSpecularColor=[0.5 0.5 0.5 1.0]  GraphicAmbientColor=[0.15 0.15 0.15 1.0]  GraphicEmissiveColor=[0.0 0.0 0.0 1.0]  GraphicShininess=75  GraphicOpacity=1
  F : PMIOPort  Side=Left
  connections:
  Solid/RConn1 -- ReferenceFrame/RConn1 -- F/RConn1

== system multi_rotor_sim/3D_visualization/SIMECHANICS 3D SCENE/SimMechanics/Assembly_Quadrotor_NProp_1_RIGID/Assembly_Quadrotor_NoProp_1_RIGID/socket_head_cap_screw_iso_17_RIGID ==
  ReferenceFrame : sm_lib/Frames and Transforms/Reference Frame
  Solid : sm_lib/Body Elements/File Solid  ExtGeomFileName=socket head cap screw_iso_ISO 4762 M3 x 5 --- 5N_sldprt.STL  UnitType=Custom  ExtGeomFileUnits=mm  StepReaderType=HEX  ExportConvexHullGeometry=off  InertiaType=Custom  Mass=9.7562055451047927e-05  MassUnits=kg  CenterOfMass=[2.9922591429378405 0 0]  CenterOfMassUnits=mm  MomentsOfInertia=[0.00030067681878230242 0.000604867911685519 0.00060486791168551911]  MomentsOfInertiaUnits=kg*mm^2  ProductsOfInertia=[0 0 0]  ProductsOfInertiaUnits=kg*mm^2  BasedOnType=Density  Density=1000  DensityUnits=kg/(m^3)  DoExposeReferenceFrame=on  SerializedFrames=<Frames/>  GraphicType=FromGeometry  MarkerShape=Sphere  MarkerSize=10  MarkerSizeUnits=m  GraphicVisPropType=SimpleVisualProperties  GraphicDiffuseColor=[0.77647058823529413 0.75686274509803919 0.73725490196078436]  GraphicSpecularColor=[0.5 0.5 0.5 1.0]  GraphicAmbientColor=[0.15 0.15 0.15 1.0]  GraphicEmissiveColor=[0.0 0.0 0.0 1.0]  GraphicShininess=75  GraphicOpacity=1
  F : PMIOPort  Side=Left
  connections:
  Solid/RConn1 -- ReferenceFrame/RConn1 -- F/RConn1

== system multi_rotor_sim/3D_visualization/SIMECHANICS 3D SCENE/SimMechanics/Assembly_Quadrotor_NProp_1_RIGID/Assembly_Quadrotor_NoProp_1_RIGID/socket_head_cap_screw_iso_18_RIGID ==
  ReferenceFrame : sm_lib/Frames and Transforms/Reference Frame
  Solid : sm_lib/Body Elements/File Solid  ExtGeomFileName=socket head cap screw_iso_ISO 4762 M3 x 5 --- 5N_sldprt.STL  UnitType=Custom  ExtGeomFileUnits=mm  StepReaderType=HEX  ExportConvexHullGeometry=off  InertiaType=Custom  Mass=9.7562055451047927e-05  MassUnits=kg  CenterOfMass=[2.9922591429378405 0 0]  CenterOfMassUnits=mm  MomentsOfInertia=[0.00030067681878230242 0.000604867911685519 0.00060486791168551911]  MomentsOfInertiaUnits=kg*mm^2  ProductsOfInertia=[0 0 0]  ProductsOfInertiaUnits=kg*mm^2  BasedOnType=Density  Density=1000  DensityUnits=kg/(m^3)  DoExposeReferenceFrame=on  SerializedFrames=<Frames/>  GraphicType=FromGeometry  MarkerShape=Sphere  MarkerSize=10  MarkerSizeUnits=m  GraphicVisPropType=SimpleVisualProperties  GraphicDiffuseColor=[0.77647058823529413 0.75686274509803919 0.73725490196078436]  GraphicSpecularColor=[0.5 0.5 0.5 1.0]  GraphicAmbientColor=[0.15 0.15 0.15 1.0]  GraphicEmissiveColor=[0.0 0.0 0.0 1.0]  GraphicShininess=75  GraphicOpacity=1
  F : PMIOPort  Side=Left
  connections:
  Solid/RConn1 -- ReferenceFrame/RConn1 -- F/RConn1

== system multi_rotor_sim/3D_visualization/SIMECHANICS 3D SCENE/SimMechanics/Assembly_Quadrotor_NProp_1_RIGID/Assembly_Quadrotor_NoProp_1_RIGID/socket_head_cap_screw_iso_19_RIGID ==
  ReferenceFrame : sm_lib/Frames and Transforms/Reference Frame
  Solid : sm_lib/Body Elements/File Solid  ExtGeomFileName=socket head cap screw_iso_ISO 4762 M3 x 5 --- 5N_sldprt.STL  UnitType=Custom  ExtGeomFileUnits=mm  StepReaderType=HEX  ExportConvexHullGeometry=off  InertiaType=Custom  Mass=9.7562055451047927e-05  MassUnits=kg  CenterOfMass=[2.9922591429378405 0 0]  CenterOfMassUnits=mm  MomentsOfInertia=[0.00030067681878230242 0.000604867911685519 0.00060486791168551911]  MomentsOfInertiaUnits=kg*mm^2  ProductsOfInertia=[0 0 0]  ProductsOfInertiaUnits=kg*mm^2  BasedOnType=Density  Density=1000  DensityUnits=kg/(m^3)  DoExposeReferenceFrame=on  SerializedFrames=<Frames/>  GraphicType=FromGeometry  MarkerShape=Sphere  MarkerSize=10  MarkerSizeUnits=m  GraphicVisPropType=SimpleVisualProperties  GraphicDiffuseColor=[0.77647058823529413 0.75686274509803919 0.73725490196078436]  GraphicSpecularColor=[0.5 0.5 0.5 1.0]  GraphicAmbientColor=[0.15 0.15 0.15 1.0]  GraphicEmissiveColor=[0.0 0.0 0.0 1.0]  GraphicShininess=75  GraphicOpacity=1
  F : PMIOPort  Side=Left
  connections:
  Solid/RConn1 -- ReferenceFrame/RConn1 -- F/RConn1

== system multi_rotor_sim/3D_visualization/SIMECHANICS 3D SCENE/SimMechanics/Assembly_Quadrotor_NProp_1_RIGID/Assembly_Quadrotor_NoProp_1_RIGID/socket_head_cap_screw_iso_20_RIGID ==
  ReferenceFrame : sm_lib/Frames and Transforms/Reference Frame
  Solid : sm_lib/Body Elements/File Solid  ExtGeomFileName=socket head cap screw_iso_ISO 4762 M3 x 5 --- 5N_sldprt.STL  UnitType=Custom  ExtGeomFileUnits=mm  StepReaderType=HEX  ExportConvexHullGeometry=off  InertiaType=Custom  Mass=9.7562055451047927e-05  MassUnits=kg  CenterOfMass=[2.9922591429378405 0 0]  CenterOfMassUnits=mm  MomentsOfInertia=[0.00030067681878230242 0.000604867911685519 0.00060486791168551911]  MomentsOfInertiaUnits=kg*mm^2  ProductsOfInertia=[0 0 0]  ProductsOfInertiaUnits=kg*mm^2  BasedOnType=Density  Density=1000  DensityUnits=kg/(m^3)  DoExposeReferenceFrame=on  SerializedFrames=<Frames/>  GraphicType=FromGeometry  MarkerShape=Sphere  MarkerSize=10  MarkerSizeUnits=m  GraphicVisPropType=SimpleVisualProperties  GraphicDiffuseColor=[0.77647058823529413 0.75686274509803919 0.73725490196078436]  GraphicSpecularColor=[0.5 0.5 0.5 1.0]  GraphicAmbientColor=[0.15 0.15 0.15 1.0]  GraphicEmissiveColor=[0.0 0.0 0.0 1.0]  GraphicShininess=75  GraphicOpacity=1
  F : PMIOPort  Side=Left
  connections:
  Solid/RConn1 -- ReferenceFrame/RConn1 -- F/RConn1

== system multi_rotor_sim/3D_visualization/SIMECHANICS 3D SCENE/SimMechanics/Assembly_Quadrotor_NProp_1_RIGID/Assembly_Quadrotor_NoProp_1_RIGID/socket_head_cap_screw_iso_21_RIGID ==
  ReferenceFrame : sm_lib/Frames and Transforms/Reference Frame
  Solid : sm_lib/Body Elements/File Solid  ExtGeomFileName=socket head cap screw_iso_ISO 4762 M3 x 5 --- 5N_sldprt.STL  UnitType=Custom  ExtGeomFileUnits=mm  StepReaderType=HEX  ExportConvexHullGeometry=off  InertiaType=Custom  Mass=9.7562055451047927e-05  MassUnits=kg  CenterOfMass=[2.9922591429378405 0 0]  CenterOfMassUnits=mm  MomentsOfInertia=[0.00030067681878230242 0.000604867911685519 0.00060486791168551911]  MomentsOfInertiaUnits=kg*mm^2  ProductsOfInertia=[0 0 0]  ProductsOfInertiaUnits=kg*mm^2  BasedOnType=Density  Density=1000  DensityUnits=kg/(m^3)  DoExposeReferenceFrame=on  SerializedFrames=<Frames/>  GraphicType=FromGeometry  MarkerShape=Sphere  MarkerSize=10  MarkerSizeUnits=m  GraphicVisPropType=SimpleVisualProperties  GraphicDiffuseColor=[0.77647058823529413 0.75686274509803919 0.73725490196078436]  GraphicSpecularColor=[0.5 0.5 0.5 1.0]  GraphicAmbientColor=[0.15 0.15 0.15 1.0]  GraphicEmissiveColor=[0.0 0.0 0.0 1.0]  GraphicShininess=75  GraphicOpacity=1
  F : PMIOPort  Side=Left
  connections:
  Solid/RConn1 -- ReferenceFrame/RConn1 -- F/RConn1

== system multi_rotor_sim/3D_visualization/SIMECHANICS 3D SCENE/SimMechanics/Assembly_Quadrotor_NProp_1_RIGID/Assembly_Quadrotor_NoProp_1_RIGID/socket_head_cap_screw_iso_22_RIGID ==
  ReferenceFrame : sm_lib/Frames and Transforms/Reference Frame
  Solid : sm_lib/Body Elements/File Solid  ExtGeomFileName=socket head cap screw_iso_ISO 4762 M3 x 5 --- 5N_sldprt.STL  UnitType=Custom  ExtGeomFileUnits=mm  StepReaderType=HEX  ExportConvexHullGeometry=off  InertiaType=Custom  Mass=9.7562055451047927e-05  MassUnits=kg  CenterOfMass=[2.9922591429378405 0 0]  CenterOfMassUnits=mm  MomentsOfInertia=[0.00030067681878230242 0.000604867911685519 0.00060486791168551911]  MomentsOfInertiaUnits=kg*mm^2  ProductsOfInertia=[0 0 0]  ProductsOfInertiaUnits=kg*mm^2  BasedOnType=Density  Density=1000  DensityUnits=kg/(m^3)  DoExposeReferenceFrame=on  SerializedFrames=<Frames/>  GraphicType=FromGeometry  MarkerShape=Sphere  MarkerSize=10  MarkerSizeUnits=m  GraphicVisPropType=SimpleVisualProperties  GraphicDiffuseColor=[0.77647058823529413 0.75686274509803919 0.73725490196078436]  GraphicSpecularColor=[0.5 0.5 0.5 1.0]  GraphicAmbientColor=[0.15 0.15 0.15 1.0]  GraphicEmissiveColor=[0.0 0.0 0.0 1.0]  GraphicShininess=75  GraphicOpacity=1
  F : PMIOPort  Side=Left
  connections:
  Solid/RConn1 -- ReferenceFrame/RConn1 -- F/RConn1

== system multi_rotor_sim/3D_visualization/SIMECHANICS 3D SCENE/SimMechanics/Assembly_Quadrotor_NProp_1_RIGID/Assembly_Quadrotor_NoProp_1_RIGID/socket_head_cap_screw_iso_23_RIGID ==
  ReferenceFrame : sm_lib/Frames and Transforms/Reference Frame
  Solid : sm_lib/Body Elements/File Solid  ExtGeomFileName=socket head cap screw_iso_ISO 4762 M3 x 5 --- 5N_sldprt.STL  UnitType=Custom  ExtGeomFileUnits=mm  StepReaderType=HEX  ExportConvexHullGeometry=off  InertiaType=Custom  Mass=9.7562055451047927e-05  MassUnits=kg  CenterOfMass=[2.9922591429378405 0 0]  CenterOfMassUnits=mm  MomentsOfInertia=[0.00030067681878230242 0.000604867911685519 0.00060486791168551911]  MomentsOfInertiaUnits=kg*mm^2  ProductsOfInertia=[0 0 0]  ProductsOfInertiaUnits=kg*mm^2  BasedOnType=Density  Density=1000  DensityUnits=kg/(m^3)  DoExposeReferenceFrame=on  SerializedFrames=<Frames/>  GraphicType=FromGeometry  MarkerShape=Sphere  MarkerSize=10  MarkerSizeUnits=m  GraphicVisPropType=SimpleVisualProperties  GraphicDiffuseColor=[0.77647058823529413 0.75686274509803919 0.73725490196078436]  GraphicSpecularColor=[0.5 0.5 0.5 1.0]  GraphicAmbientColor=[0.15 0.15 0.15 1.0]  GraphicEmissiveColor=[0.0 0.0 0.0 1.0]  GraphicShininess=75  GraphicOpacity=1
  F : PMIOPort  Side=Left
  connections:
  Solid/RConn1 -- ReferenceFrame/RConn1 -- F/RConn1

== system multi_rotor_sim/3D_visualization/SIMECHANICS 3D SCENE/SimMechanics/Assembly_Quadrotor_NProp_1_RIGID/Assembly_Quadrotor_NoProp_1_RIGID/socket_head_cap_screw_iso_24_RIGID ==
  ReferenceFrame : sm_lib/Frames and Transforms/Reference Frame
  Solid : sm_lib/Body Elements/File Solid  ExtGeomFileName=socket head cap screw_iso_ISO 4762 M3 x 5 --- 5N_sldprt.STL  UnitType=Custom  ExtGeomFileUnits=mm  StepReaderType=HEX  ExportConvexHullGeometry=off  InertiaType=Custom  Mass=9.7562055451047927e-05  MassUnits=kg  CenterOfMass=[2.9922591429378405 0 0]  CenterOfMassUnits=mm  MomentsOfInertia=[0.00030067681878230242 0.000604867911685519 0.00060486791168551911]  MomentsOfInertiaUnits=kg*mm^2  ProductsOfInertia=[0 0 0]  ProductsOfInertiaUnits=kg*mm^2  BasedOnType=Density  Density=1000  DensityUnits=kg/(m^3)  DoExposeReferenceFrame=on  SerializedFrames=<Frames/>  GraphicType=FromGeometry  MarkerShape=Sphere  MarkerSize=10  MarkerSizeUnits=m  GraphicVisPropType=SimpleVisualProperties  GraphicDiffuseColor=[0.77647058823529413 0.75686274509803919 0.73725490196078436]  GraphicSpecularColor=[0.5 0.5 0.5 1.0]  GraphicAmbientColor=[0.15 0.15 0.15 1.0]  GraphicEmissiveColor=[0.0 0.0 0.0 1.0]  GraphicShininess=75  GraphicOpacity=1
  F : PMIOPort  Side=Left
  connections:
  Solid/RConn1 -- ReferenceFrame/RConn1 -- F/RConn1

== system multi_rotor_sim/3D_visualization/SIMECHANICS 3D SCENE/SimMechanics/Assembly_Quadrotor_NProp_1_RIGID/Assembly_Quadrotor_NoProp_1_RIGID/socket_head_cap_screw_iso_25_RIGID ==
  ReferenceFrame : sm_lib/Frames and Transforms/Reference Frame
  Solid : sm_lib/Body Elements/File Solid  ExtGeomFileName=socket head cap screw_iso_ISO 4762 M3 x 5 --- 5N_sldprt.STL  UnitType=Custom  ExtGeomFileUnits=mm  StepReaderType=HEX  ExportConvexHullGeometry=off  InertiaType=Custom  Mass=9.7562055451047927e-05  MassUnits=kg  CenterOfMass=[2.9922591429378405 0 0]  CenterOfMassUnits=mm  MomentsOfInertia=[0.00030067681878230242 0.000604867911685519 0.00060486791168551911]  MomentsOfInertiaUnits=kg*mm^2  ProductsOfInertia=[0 0 0]  ProductsOfInertiaUnits=kg*mm^2  BasedOnType=Density  Density=1000  DensityUnits=kg/(m^3)  DoExposeReferenceFrame=on  SerializedFrames=<Frames/>  GraphicType=FromGeometry  MarkerShape=Sphere  MarkerSize=10  MarkerSizeUnits=m  GraphicVisPropType=SimpleVisualProperties  GraphicDiffuseColor=[0.77647058823529413 0.75686274509803919 0.73725490196078436]  GraphicSpecularColor=[0.5 0.5 0.5 1.0]  GraphicAmbientColor=[0.15 0.15 0.15 1.0]  GraphicEmissiveColor=[0.0 0.0 0.0 1.0]  GraphicShininess=75  GraphicOpacity=1
  F : PMIOPort  Side=Left
  connections:
  Solid/RConn1 -- ReferenceFrame/RConn1 -- F/RConn1

== system multi_rotor_sim/3D_visualization/SIMECHANICS 3D SCENE/SimMechanics/Assembly_Quadrotor_NProp_1_RIGID/Assembly_Quadrotor_NoProp_1_RIGID/socket_head_cap_screw_iso_2_RIGID ==
  ReferenceFrame : sm_lib/Frames and Transforms/Reference Frame
  Solid : sm_lib/Body Elements/File Solid  ExtGeomFileName=socket head cap screw_iso_ISO 4762 M3 x 5 --- 5N_sldprt.STL  UnitType=Custom  ExtGeomFileUnits=mm  StepReaderType=HEX  ExportConvexHullGeometry=off  InertiaType=Custom  Mass=9.7562055451047927e-05  MassUnits=kg  CenterOfMass=[2.9922591429378405 0 0]  CenterOfMassUnits=mm  MomentsOfInertia=[0.00030067681878230242 0.000604867911685519 0.00060486791168551911]  MomentsOfInertiaUnits=kg*mm^2  ProductsOfInertia=[0 0 0]  ProductsOfInertiaUnits=kg*mm^2  BasedOnType=Density  Density=1000  DensityUnits=kg/(m^3)  DoExposeReferenceFrame=on  SerializedFrames=<Frames/>  GraphicType=FromGeometry  MarkerShape=Sphere  MarkerSize=10  MarkerSizeUnits=m  GraphicVisPropType=SimpleVisualProperties  GraphicDiffuseColor=[0.77647058823529413 0.75686274509803919 0.73725490196078436]  GraphicSpecularColor=[0.5 0.5 0.5 1.0]  GraphicAmbientColor=[0.15 0.15 0.15 1.0]  GraphicEmissiveColor=[0.0 0.0 0.0 1.0]  GraphicShininess=75  GraphicOpacity=1
  F : PMIOPort  Side=Left
  connections:
  Solid/RConn1 -- ReferenceFrame/RConn1 -- F/RConn1

== system multi_rotor_sim/3D_visualization/SIMECHANICS 3D SCENE/SimMechanics/Assembly_Quadrotor_NProp_1_RIGID/Assembly_Quadrotor_NoProp_1_RIGID/socket_head_cap_screw_iso_3_RIGID ==
  ReferenceFrame : sm_lib/Frames and Transforms/Reference Frame
  Solid : sm_lib/Body Elements/File Solid  ExtGeomFileName=socket head cap screw_iso_ISO 4762 M3 x 5 --- 5N_sldprt.STL  UnitType=Custom  ExtGeomFileUnits=mm  StepReaderType=HEX  ExportConvexHullGeometry=off  InertiaType=Custom  Mass=9.7562055451047927e-05  MassUnits=kg  CenterOfMass=[2.9922591429378405 0 0]  CenterOfMassUnits=mm  MomentsOfInertia=[0.00030067681878230242 0.000604867911685519 0.00060486791168551911]  MomentsOfInertiaUnits=kg*mm^2  ProductsOfInertia=[0 0 0]  ProductsOfInertiaUnits=kg*mm^2  BasedOnType=Density  Density=1000  DensityUnits=kg/(m^3)  DoExposeReferenceFrame=on  SerializedFrames=<Frames/>  GraphicType=FromGeometry  MarkerShape=Sphere  MarkerSize=10  MarkerSizeUnits=m  GraphicVisPropType=SimpleVisualProperties  GraphicDiffuseColor=[0.77647058823529413 0.75686274509803919 0.73725490196078436]  GraphicSpecularColor=[0.5 0.5 0.5 1.0]  GraphicAmbientColor=[0.15 0.15 0.15 1.0]  GraphicEmissiveColor=[0.0 0.0 0.0 1.0]  GraphicShininess=75  GraphicOpacity=1
  F : PMIOPort  Side=Left
  connections:
  Solid/RConn1 -- ReferenceFrame/RConn1 -- F/RConn1
